simulink model "M_1"  (Simulink 7.0)
settings: Solver=ode1  StartTime=0.0  StopTime=5  FixedStep=0.0001  RelTol=1e-3
libraries: simulink x2
settings Model: Creator=student  LastModifiedBy=Dr.Alex

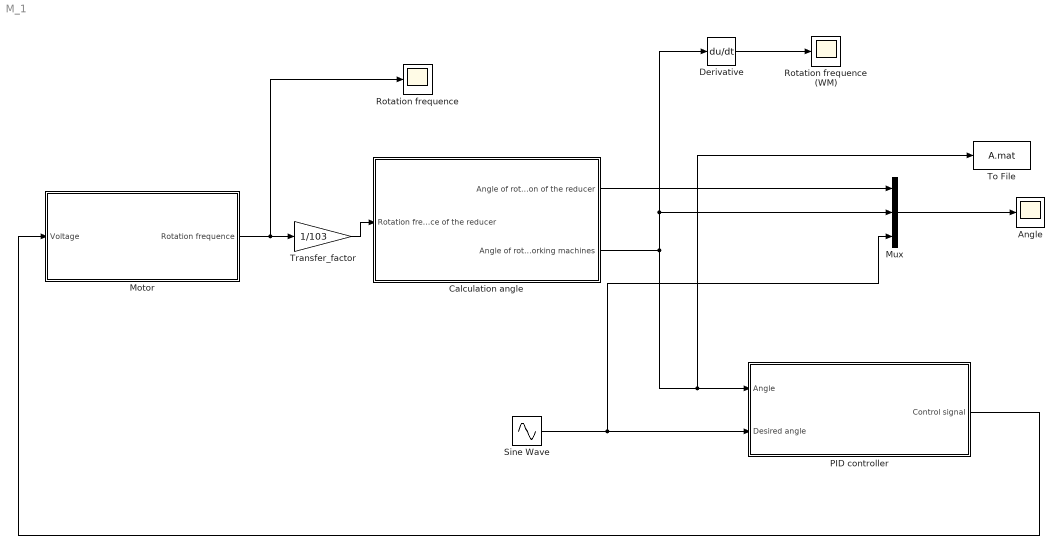
== system M_1 ==
  Angle : Scope
      settings: TimeRange=0.12  YMin=-0.48  YMax=-0.3  SaveName=ScopeData8  MaxDataPoints=300000
  Calculation angle : Subsystem
  Derivative : Derivative
  Motor : Subsystem
  Mux : Mux  Inputs=3
  PID controller : Subsystem  mask{k=100, t_i=0.04, t_d=0.01, d=1, i=1}
      mask prompts: k "Proportional gain"; t_i "Integral time"; t_d "Derivative ime"; d "Setting factor D"; i "Setting factor I"
  Rotation frequence : Scope
      settings: TimeRange=0.2  YMin=9.23979  YMax=10.2124  MaxDataPoints=150000
  Rotation frequence (WM) : Scope
      settings: TimeRange=0.2  YMin=-0.001  YMax=0.012  MaxDataPoints=150000
  Sine Wave : Sin  Amplitude=pi/180  Frequency=pi/5  SampleTime=0
  To File : ToFile  Filename=A.mat  MatrixName=a
  Transfer_factor : Gain  Gain=1/103  ParameterDataType=sfix(16)  ParameterScaling=2^0  OutDataType=sfix(16)  OutScaling=2^0
  wires:
  Motor/1(Rotation frequence) -> Transfer_factor/1, Rotation frequence/1
  Mux/1 -> Angle/1
  Transfer_factor/1 -> Calculation angle/1(Rotation frequence of the reducer)
  Sine Wave/1 -> Mux/3, PID controller/2(Desired angle)
  Calculation angle/1(Angle of rotation of the reducer) -> Mux/1
  Calculation angle/2(Angle of rotation of the working machines) -> Derivative/1, Mux/2, PID controller/1(Angle), To File/1
  Derivative/1 -> Rotation frequence (WM)/1
  PID controller/1(Control signal) -> Motor/1(Voltage)

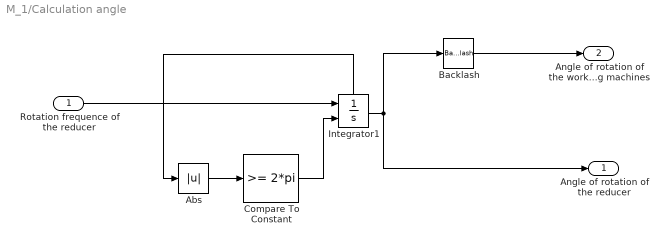
== system M_1/Calculation angle ==
  Rotation frequence of the reducer : Inport
  Abs : Abs  OutDataType=sfix(16)  OutScaling=2^0
  Backlash : Backlash  BacklashWidth=pi/180
  Compare To Constant : simulink/Logic and Bit Operations/Compare To Constant  SystemSampleTime=-1  relop=>=  const=2*pi  LogicOutDataTypeMode=boolean  ZeroCross=off
  Integrator1 : Integrator  ExternalReset=level  UpperSaturationLimit=6.28  ShowStatePort=on
  Angle of rotation of the reducer : Outport
  Angle of rotation of the working machines : Outport  Port=2
  wires:
  Integrator1/State -> Abs/1
  Compare To Constant/1 -> Integrator1/2
  Abs/1 -> Compare To Constant/1
  Integrator1/1 -> Angle of rotation of the reducer/1, Backlash/1
  Rotation frequence of the reducer/1 -> Integrator1/1
  Backlash/1 -> Angle of rotation of the working machines/1

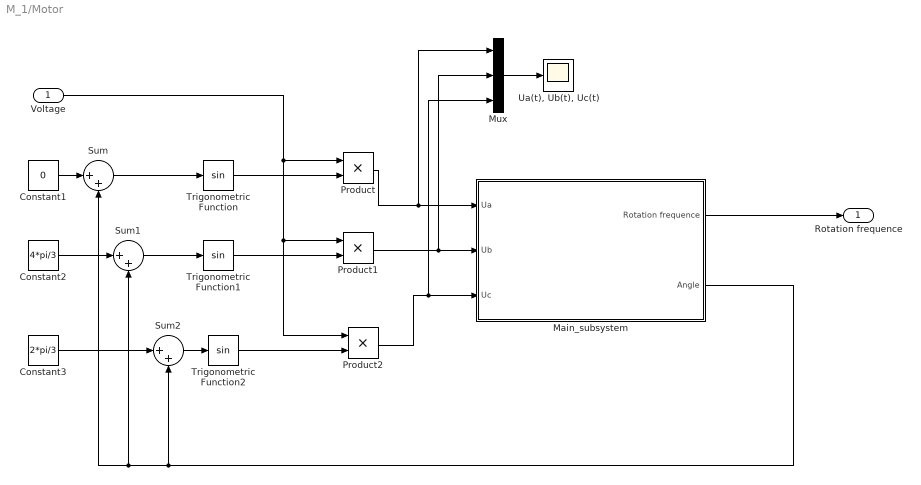
== system M_1/Motor ==
  Voltage : Inport  OutDataType=sfix(16)  OutScaling=2^0
  Constant1 : Constant  Value=0  OutDataType=sfix(16)  OutScaling=2^0
  Constant2 : Constant  Value=4*pi/3  OutDataType=sfix(16)  OutScaling=2^0
  Constant3 : Constant  Value=2*pi/3  OutDataType=sfix(16)  OutScaling=2^0
  Main_subsystem : Subsystem
  Mux : Mux  Inputs=3
  Product : Product  OutDataType=sfix(16)  OutScaling=2^0  RndMeth=Zero
  Product1 : Product  OutDataType=sfix(16)  OutScaling=2^0  RndMeth=Zero
  Product2 : Product  OutDataType=sfix(16)  OutScaling=2^0  RndMeth=Zero
  Sum : Sum  Inputs=|++  OutDataType=sfix(16)  OutScaling=2^0
  Sum1 : Sum  Inputs=|++  OutDataType=sfix(16)  OutScaling=2^0
  Sum2 : Sum  Inputs=|++  OutDataType=sfix(16)  OutScaling=2^0
  Trigonometric Function : Trigonometry
  Trigonometric Function1 : Trigonometry
  Trigonometric Function2 : Trigonometry
  "Ua(t), Ub(t), Uc(t)" : Scope
      settings: YMin=-9  YMax=9  SaveName=ScopeData2  MaxDataPoints=200000
  Rotation frequence : Outport  OutDataType=sfix(16)  OutScaling=2^0
  wires:
  Main_subsystem/1(Rotation frequence) -> Rotation frequence/1
  Main_subsystem/2(Angle) -> Sum/2, Sum1/2, Sum2/2
  Product/1 -> Main_subsystem/1(Ua), Mux/1
  Product1/1 -> Main_subsystem/2(Ub), Mux/2
  Product2/1 -> Main_subsystem/3(Uc), Mux/3
  Trigonometric Function2/1 -> Product2/2
  Trigonometric Function1/1 -> Product1/2
  Trigonometric Function/1 -> Product/2
  Voltage/1 -> Product/1, Product1/1, Product2/1
  Sum/1 -> Trigonometric Function/1
  Sum1/1 -> Trigonometric Function1/1
  Sum2/1 -> Trigonometric Function2/1
  Constant1/1 -> Sum/1
  Constant2/1 -> Sum1/1
  Constant3/1 -> Sum2/1
  Mux/1 -> "Ua(t), Ub(t), Uc(t)"/1

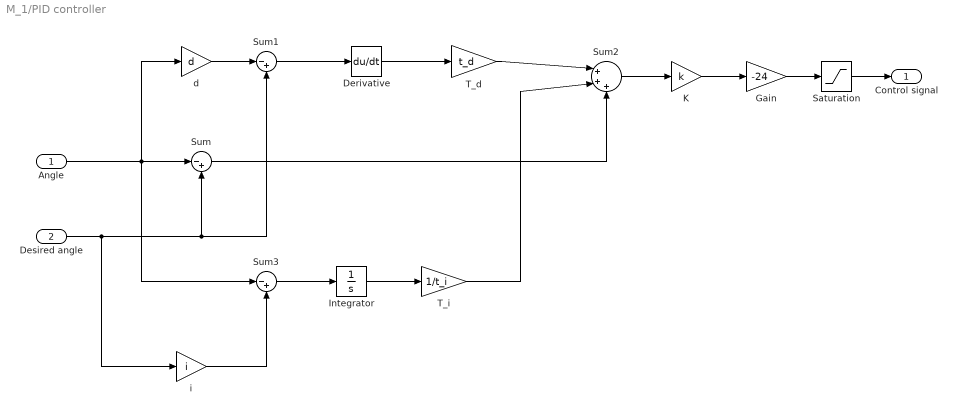
== system M_1/PID controller ==
  Angle : Inport
  Desired angle : Inport  Port=2
  Derivative : Derivative
  Gain : Gain  Gain=-24  ParameterDataType=sfix(16)  ParameterScaling=2^0  OutDataType=sfix(16)  OutScaling=2^0
  Integrator : Integrator
  K : Gain  Gain=k  ParameterDataType=sfix(16)  ParameterScaling=2^0  OutDataType=sfix(16)  OutScaling=2^0
  Saturation : Saturate  UpperLimit=24  LowerLimit=-24  OutDataType=sfix(16)  OutScaling=2^0
  Sum : Sum  Inputs=|-+  OutDataType=sfix(16)  OutScaling=2^0
  Sum1 : Sum  Inputs=|-+  OutDataType=sfix(16)  OutScaling=2^0
  Sum2 : Sum  Inputs=|+++  OutDataType=sfix(16)  OutScaling=2^0
  Sum3 : Sum  Inputs=|-+  OutDataType=sfix(16)  OutScaling=2^0
  T_d : Gain  Gain=t_d  ParameterDataType=sfix(16)  ParameterScaling=2^0  OutDataType=sfix(16)  OutScaling=2^0
  T_i : Gain  Gain=1/t_i  ParameterDataType=sfix(16)  ParameterScaling=2^0  OutDataType=sfix(16)  OutScaling=2^0
  d : Gain  Gain=d  ParameterDataType=sfix(16)  ParameterScaling=2^0  OutDataType=sfix(16)  OutScaling=2^0
  i : Gain  Gain=i  ParameterDataType=sfix(16)  ParameterScaling=2^0  OutDataType=sfix(16)  OutScaling=2^0
  Control signal : Outport
  wires:
  Desired angle/1 -> Sum/2, Sum1/2, i/1
  Angle/1 -> Sum/1, Sum3/1, d/1
  Sum2/1 -> K/1
  T_d/1 -> Sum2/1
  T_i/1 -> Sum2/2
  Integrator/1 -> T_i/1
  Sum/1 -> Sum2/3
  Gain/1 -> Saturation/1
  Saturation/1 -> Control signal/1
  Derivative/1 -> T_d/1
  Sum1/1 -> Derivative/1
  Sum3/1 -> Integrator/1
  d/1 -> Sum1/1
  i/1 -> Sum3/2
  K/1 -> Gain/1

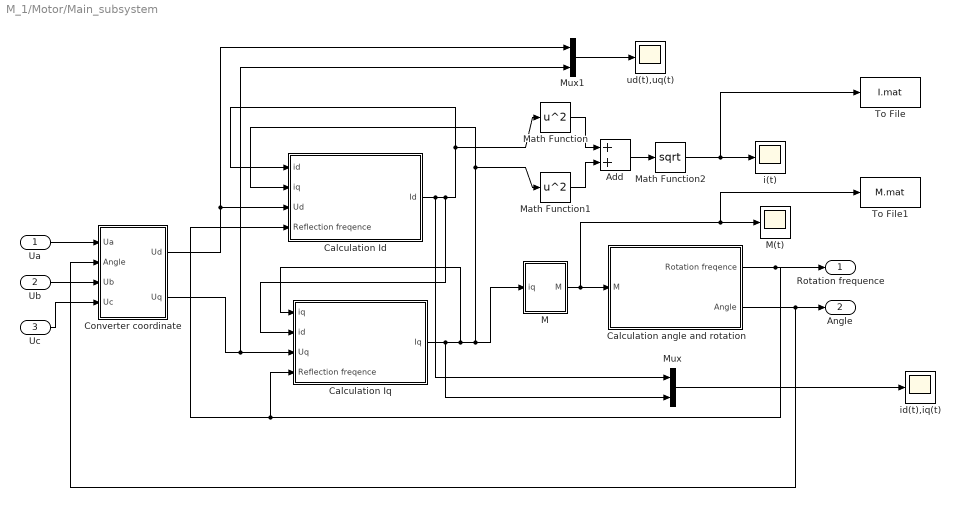
== system M_1/Motor/Main_subsystem ==
  Ua : Inport
  Ub : Inport  Port=2
  Uc : Inport  Port=3
  Add : Sum  OutDataType=sfix(16)  OutScaling=2^-10
  Calculation Id : Subsystem  mask{L=0.000226, R=1.39, p=1}
  Calculation Iq : Subsystem  mask{L=0.000226, R=1.39, p=1, F=0.02052}
  Calculation angle and rotation : Subsystem
  Converter coordinate : Subsystem
  M : Subsystem  mask{p=1, F=0.02052}
  M(t) : Scope
      settings: TimeRange=0.0009635850577801668  YMin=0.01753  YMax=0.0175775  SaveName=ScopeData4  MaxDataPoints=50000
  Math Function : Math  Operator=square  OutDataType=sfix(16)  OutScaling=2^0  SaturateOnIntegerOverflow=on
  Math Function1 : Math  Operator=square  OutDataType=sfix(16)  OutScaling=2^0  SaturateOnIntegerOverflow=on
  Math Function2 : Math  Operator=sqrt  OutDataType=sfix(16)  OutScaling=2^0  SaturateOnIntegerOverflow=on
  Mux : Mux  Inputs=2
  Mux1 : Mux  Inputs=2
  To File : ToFile  Filename=I.mat  MatrixName=I
  To File1 : ToFile  Filename=M.mat  MatrixName=M
  i(t) : Scope
      settings: TimeRange=0.02049180327868855  YMin=1.0815e-012  YMax=1.08675e-012  SaveName=ScopeData3  MaxDataPoints=50000
  id(t),iq(t) : Scope
      settings: TimeRange=0.0001335326525127652  YMin=0.6  YMax=2.4  SaveName=ScopeData5  MaxDataPoints=50000
  ud(t),uq(t) : Scope
      settings: TimeRange=0.0001335326525127652  YMin=0.6  YMax=2.4  SaveName=ScopeData7  MaxDataPoints=50000
  Rotation frequence : Outport
  Angle : Outport  Port=2  OutDataType=sfix(16)  OutScaling=2^0
  wires:
  Calculation angle and rotation/1(Rotation freqence) -> Rotation frequence/1, Calculation Iq/4(Reflection freqence), Calculation Id/4(Reflection freqence)
  Ua/1 -> Converter coordinate/1(Ua)
  Calculation angle and rotation/2(Angle) -> Angle/1, Converter coordinate/2(Angle)
  M/1(M) -> Calculation angle and rotation/1(M), M(t)/1, To File1/1
  Uc/1 -> Converter coordinate/4(Uc)
  Ub/1 -> Converter coordinate/3(Ub)
  Calculation Id/1(Id) -> Calculation Iq/2(id), Calculation Id/1(id), Math Function/1, Mux/1
  Converter coordinate/2(Uq) -> Calculation Iq/3(Uq), Mux1/2
  Converter coordinate/1(Ud) -> Calculation Id/3(Ud), Mux1/1
  Calculation Iq/1(Iq) -> Calculation Id/2(iq), Math Function1/1, M/1(iq), Calculation Iq/1(iq), Mux/2
  Math Function/1 -> Add/1
  Math Function1/1 -> Add/2
  Add/1 -> Math Function2/1
  Math Function2/1 -> i(t)/1, To File/1
  Mux/1 -> id(t),iq(t)/1
  Mux1/1 -> ud(t),uq(t)/1

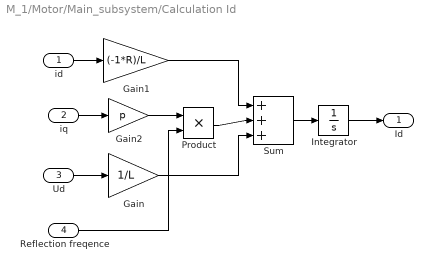
== system M_1/Motor/Main_subsystem/Calculation Id ==
  id : Inport  OutDataType=sfix(16)  OutScaling=2^0
  iq : Inport  Port=2  OutDataType=sfix(16)  OutScaling=2^0
  Ud : Inport  Port=3  OutDataType=sfix(16)  OutScaling=2^0
  Reflection freqence : Inport  Port=4  OutDataType=sfix(16)  OutScaling=2^0
  Gain : Gain  Gain=1/L  ParameterDataType=sfix(16)  ParameterScaling=2^0  OutDataType=sfix(16)  OutScaling=2^0
  Gain1 : Gain  Gain=(-1*R)/L  ParameterDataType=sfix(16)  ParameterScaling=2^0  OutDataType=sfix(16)  OutScaling=2^0
  Gain2 : Gain  Gain=p  ParameterDataType=sfix(16)  ParameterScaling=2^0  OutDataType=sfix(16)  OutScaling=2^0
  Integrator : Integrator
  Product : Product  OutDataType=sfix(16)  OutScaling=2^0  RndMeth=Zero
  Sum : Sum  Inputs=|+++  OutDataType=sfix(16)  OutScaling=2^0
  Id : Outport  OutDataType=sfix(16)  OutScaling=2^0
  wires:
  Ud/1 -> Gain/1
  id/1 -> Gain1/1
  Reflection freqence/1 -> Product/2
  Gain1/1 -> Sum/1
  Product/1 -> Sum/2
  Gain/1 -> Sum/3
  Sum/1 -> Integrator/1
  Integrator/1 -> Id/1
  iq/1 -> Gain2/1
  Gain2/1 -> Product/1

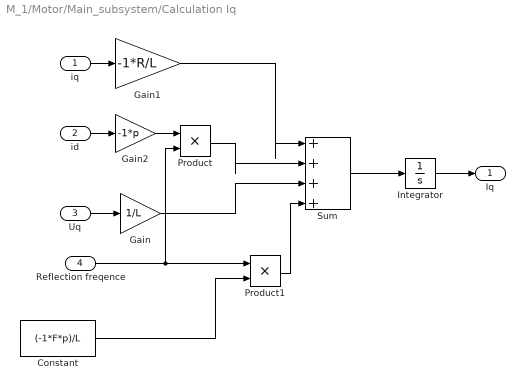
== system M_1/Motor/Main_subsystem/Calculation Iq ==
  iq : Inport  OutDataType=sfix(16)  OutScaling=2^0
  id : Inport  Port=2  OutDataType=sfix(16)  OutScaling=2^0
  Uq : Inport  Port=3  OutDataType=sfix(16)  OutScaling=2^0
  Reflection freqence : Inport  Port=4  OutDataType=sfix(16)  OutScaling=2^0
  Constant : Constant  Value=(-1*F*p)/L  OutDataType=sfix(16)  OutScaling=2^0
  Gain : Gain  Gain=1/L  ParameterDataType=sfix(16)  ParameterScaling=2^0  OutDataType=sfix(16)  OutScaling=2^0
  Gain1 : Gain  Gain=-1*R/L  ParameterDataType=sfix(16)  ParameterScaling=2^0  OutDataType=sfix(16)  OutScaling=2^0
  Gain2 : Gain  Gain=-1*p  ParameterDataType=sfix(16)  ParameterScaling=2^0  OutDataType=sfix(16)  OutScaling=2^0
  Integrator : Integrator
  Product : Product  OutDataType=sfix(16)  OutScaling=2^0  RndMeth=Zero
  Product1 : Product  OutDataType=sfix(16)  OutScaling=2^0  RndMeth=Zero
  Sum : Sum  Inputs=|++++  OutDataType=sfix(16)  OutScaling=2^0
  Iq : Outport  OutDataType=sfix(16)  OutScaling=2^0
  wires:
  Uq/1 -> Gain/1
  iq/1 -> Gain1/1
  Gain2/1 -> Product/1
  Reflection freqence/1 -> Product1/1, Product/2
  Gain1/1 -> Sum/1
  Product/1 -> Sum/2
  Gain/1 -> Sum/3
  Sum/1 -> Integrator/1
  Integrator/1 -> Iq/1
  id/1 -> Gain2/1
  Constant/1 -> Product1/2
  Product1/1 -> Sum/4

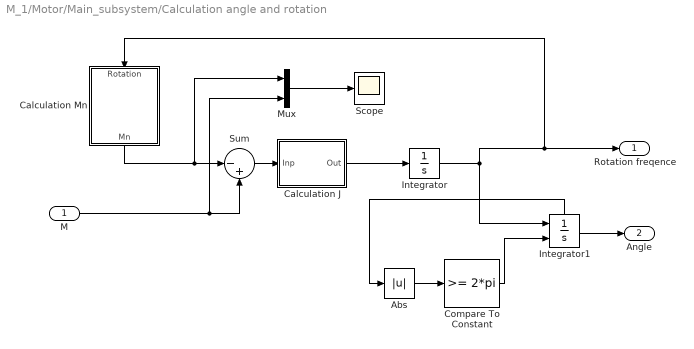
== system M_1/Motor/Main_subsystem/Calculation angle and rotation ==
  M : Inport
  Abs : Abs  OutDataType=sfix(16)  OutScaling=2^0
  Calculation J : Subsystem  mask{J0=0.0000020, J1=0.00000007, J2=0, k_r=103, n_r=0.7}
      mask prompts: J0 "The moment of inertia of the working machine"; J1 "The moment of inertia of the reducer"; J2 "The moment of inertia of the working machine"; k_r "Gear ratio of the reducer"; n_r "Efficiency of the reducer"
  Calculation Mn : Subsystem  Orientation=down  mask{M0=0.00639, M1=0, M2=0, k_r=103, n_r=0.7}
      mask prompts: M0 "The moment of resistance of the engine"; M1 "The moment of resistance of the reducer"; M2 "The moment of resistance of the working machine"; k_r "Gear ratio of the reducer"; n_r "Efficiency of the reducer"
  Compare To Constant : simulink/Logic and Bit Operations/Compare To Constant  SystemSampleTime=-1  relop=>=  const=2*pi  LogicOutDataTypeMode=boolean  ZeroCross=off
  Integrator : Integrator
  Integrator1 : Integrator  ExternalReset=level  UpperSaturationLimit=6.28  ShowStatePort=on
  Mux : Mux  Inputs=2
  Scope : Scope
      settings: YMin=-0.06  YMax=-0.005  SaveName=ScopeData6
  Sum : Sum  Inputs=|-+  OutDataType=sfix(16)  OutScaling=2^0
  Rotation freqence : Outport  OutDataType=sfix(16)  OutScaling=2^0
  Angle : Outport  Port=2  OutDataType=sfix(16)  OutScaling=2^0
  wires:
  Calculation J/1(Out) -> Integrator/1
  Integrator/1 -> Integrator1/1, Rotation freqence/1, Calculation Mn/1(Rotation)
  Integrator1/1 -> Angle/1
  Integrator1/State -> Abs/1
  Compare To Constant/1 -> Integrator1/2
  Abs/1 -> Compare To Constant/1
  Sum/1 -> Calculation J/1(Inp)
  Calculation Mn/1(Mn) -> Sum/1, Mux/1
  M/1 -> Sum/2, Mux/2
  Mux/1 -> Scope/1

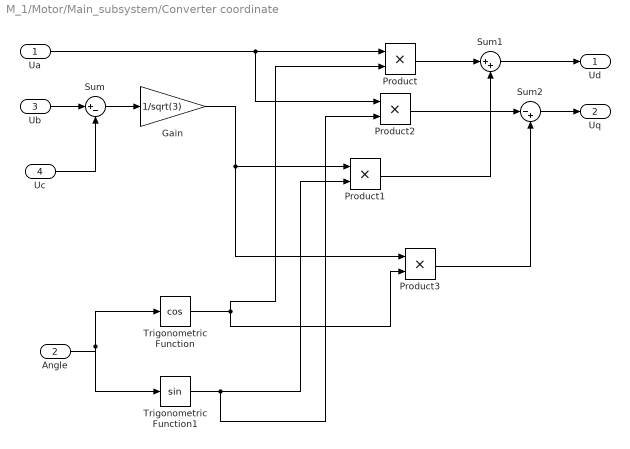
== system M_1/Motor/Main_subsystem/Converter coordinate ==
  Ua : Inport
  Angle : Inport  Port=2  OutDataType=sfix(16)  OutScaling=2^0
  Ub : Inport  Port=3  OutDataType=sfix(16)  OutScaling=2^0
  Uc : Inport  Port=4  OutDataType=sfix(16)  OutScaling=2^0
  Gain : Gain  Gain=1/sqrt(3)  ParameterDataType=sfix(16)  ParameterScaling=2^0  OutDataType=sfix(16)  OutScaling=2^0
  Product{,1..3} (4 alike) : Product  OutDataType=sfix(16)  OutScaling=2^0  RndMeth=Zero
  Sum : Sum  Inputs=|+-  OutDataType=sfix(16)  OutScaling=2^0
  Sum1 : Sum  Inputs=|++  OutDataType=sfix(16)  OutScaling=2^0
  Sum2 : Sum  Inputs=|-+  OutDataType=sfix(16)  OutScaling=2^0
  Trigonometric Function : Trigonometry  Operator=cos
  Trigonometric Function1 : Trigonometry
  Ud : Outport  OutDataType=sfix(16)  OutScaling=2^0
  Uq : Outport  Port=2  OutDataType=sfix(16)  OutScaling=2^0
  wires:
  Product/1 -> Sum1/1
  Product1/1 -> Sum1/2
  Product2/1 -> Sum2/1
  Product3/1 -> Sum2/2
  Angle/1 -> Trigonometric Function/1, Trigonometric Function1/1
  Trigonometric Function/1 -> Product3/2, Product/2
  Trigonometric Function1/1 -> Product2/2, Product1/2
  Sum1/1 -> Ud/1
  Sum2/1 -> Uq/1
  Sum/1 -> Gain/1
  Ub/1 -> Sum/1
  Uc/1 -> Sum/2
  Ua/1 -> Product/1, Product2/1
  Gain/1 -> Product1/1, Product3/1

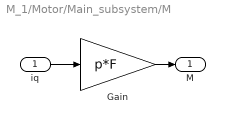
== system M_1/Motor/Main_subsystem/M ==
  iq : Inport
  Gain : Gain  Gain=p*F  ParameterDataType=sfix(16)  ParameterScaling=2^0  OutDataType=sfix(16)  OutScaling=2^0
  M : Outport  OutDataType=sfix(16)  OutScaling=2^0
  wires:
  Gain/1 -> M/1
  iq/1 -> Gain/1

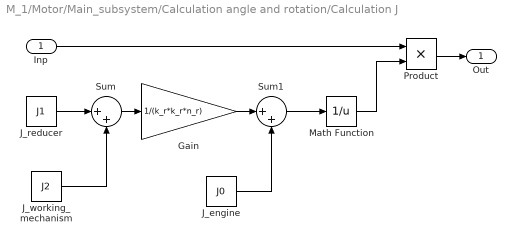
== system M_1/Motor/Main_subsystem/Calculation angle and rotation/Calculation J ==
  Inp : Inport
  Gain : Gain  Gain=1/(k_r*k_r*n_r)  ParameterDataType=sfix(16)  ParameterScaling=2^0  OutDataType=sfix(16)  OutScaling=2^0
  J_engine : Constant  Value=J0  OutDataType=sfix(16)  OutScaling=2^0
  J_reducer : Constant  Value=J1  OutDataType=sfix(16)  OutScaling=2^0
  J_working_mechanism : Constant  Value=J2  OutDataType=sfix(16)  OutScaling=2^0
  Math Function : Math  Operator=reciprocal  OutDataType=sfix(16)  OutScaling=2^0  SaturateOnIntegerOverflow=on
  Product : Product  OutDataType=sfix(16)  OutScaling=2^0  RndMeth=Zero
  Sum : Sum  Inputs=|++  OutDataType=sfix(16)  OutScaling=2^0
  Sum1 : Sum  Inputs=|++  OutDataType=sfix(16)  OutScaling=2^0
  Out : Outport
  wires:
  Sum/1 -> Gain/1
  Product/1 -> Out/1
  Inp/1 -> Product/1
  Math Function/1 -> Product/2
  J_reducer/1 -> Sum/1
  J_working_mechanism/1 -> Sum/2
  Gain/1 -> Sum1/1
  Sum1/1 -> Math Function/1
  J_engine/1 -> Sum1/2

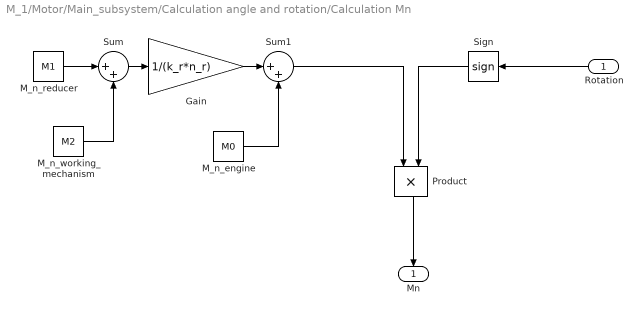
== system M_1/Motor/Main_subsystem/Calculation angle and rotation/Calculation Mn ==
  Rotation : Inport  Orientation=left
  Gain : Gain  Gain=1/(k_r*n_r)  ParameterDataType=sfix(16)  ParameterScaling=2^0  OutDataType=sfix(16)  OutScaling=2^0
  M_n_engine : Constant  Value=M0  OutDataType=sfix(16)  OutScaling=2^0
  M_n_reducer : Constant  Value=M1  OutDataType=sfix(16)  OutScaling=2^0
  M_n_working_mechanism : Constant  Value=M2  OutDataType=sfix(16)  OutScaling=2^0
  Product : Product  Orientation=down  OutDataType=sfix(16)  OutScaling=2^0  RndMeth=Zero
  Sign : Signum  Orientation=left
  Sum : Sum  Inputs=|++  OutDataType=sfix(16)  OutScaling=2^0
  Sum1 : Sum  Inputs=|++  OutDataType=sfix(16)  OutScaling=2^0
  Mn : Outport  Orientation=down
  wires:
  Rotation/1 -> Sign/1
  Sum/1 -> Gain/1
  M_n_reducer/1 -> Sum/1
  M_n_working_mechanism/1 -> Sum/2
  Gain/1 -> Sum1/1
  Sum1/1 -> Product/1
  M_n_engine/1 -> Sum1/2
  Sign/1 -> Product/2
  Product/1 -> Mn/1
